simulink model "Control_v2"  (R2019b)
settings: Solver=FixedStepAuto  StartTime=0.0  StopTime=10  FixedStep=str2num(Step_size)  RelTol=1e-3
model workspace: external: MATLAB File H:\4-project\matlab\github\Sim-v2\bicopter_sim\Bicopter_DataFile14.m (data not in the file)
values from neighbouring files (symbols this model uses):
  b = [5,1,5,4]    [init_ADRC_val.m]    (also in init_Non_Linear_ADRC_val.m = 0.5*[1,    1, 6,  6]')
  b_sep = gains(5:8)    [get_ADRC_parameters.m]    (also in get_adrc_sep.m = [  2   7    6   7]; get_adrc_sep_kalman.m = [  2   2    6   7])
  C = [eye(4),zeros(4,8)]    [init_ADRC_val.m]
  C_air = 0.0025    [Sim_Script.m]
  d_f_phi = 100    [Sim_Script.m]
  d_f_psi = 25    [Sim_Script.m]
  d_f_theta = 10    [Sim_Script.m]
  d_f_z = 100    [Sim_Script.m]
  eps_sep = 0.7*[1 1 1 1]    [get_ADRC_parameters.m]    (also in get_adrc_sep.m = [0.7 0.3 0.3 0.35]; get_adrc_sep_kalman.m = [0.7 0.7 0.3 0.35])
  epsi = 1.5    [init_Non_Linear_ADRC_val.m]
  euler_source = 1    [Sim_Script.m]
  freq_cut_angvel_phi = 75    [Sim_Script.m]
  freq_cut_angvel_psi = 75    [Sim_Script.m]
  freq_cut_angvel_theta = 50    [Sim_Script.m]
  g = 9.81    [Sim_Script.m]
  K = place(A1,B1,w00(1:8))    [init_ADRC_val.m]
  L = place(A',C',8*w00)'    [init_ADRC_val.m]
  method = STSC_controller    (= 2)    [Sim_Script.m]
  method_angle_plane_sw = plane_sw    (= 2)    [Sim_Script.m]
  mult_obs = 10    [init_Non_Linear_ADRC_val.m]
  Noise_gain = 1    [Sim_Script.m]
  PID_VAL_SEP = init_pid_val_sep()    [Sim_Script.m]
  polarity = [-1;1;1;1]    [Sim_Script.m]
  r = [10,5,10,10]    [init_Non_Linear_ADRC_val.m]
  S_phi = 0.001    [Sim_Script.m]
  S_psi = S_phi    (= 0.001)    [Sim_Script.m]
  S_theta = S_phi    (= 0.001)    [Sim_Script.m]
  State_step = [Z_step;Phi_step;Theta_step;Psi_step]    [req_response.m]
  Step_size = step_size    [Sim_Script.m]
  STSC_VAL = init_STSC_val()    [Sim_Script.m]
  time_delay = 1e-6    (= 1e-06)    [Sim_Script.m]
  V_phi = 0.01    [Sim_Script.m]
  V_psi = 0.01    [Sim_Script.m]
  V_theta = 0.01    [Sim_Script.m]
  wc_sep = gains(1:4)    [get_ADRC_parameters.m]    (also in get_adrc_sep.m = [ 5.54   9   6    3]; get_adrc_sep_kalman.m = [ 5.54   9   6    3])
  wo_sep = ga*wc_sep    [get_ADRC_parameters.m]    (also in get_adrc_sep.m; get_adrc_sep_kalman.m)
undefined symbols (not defined in the file or in its folder): Continuous, magnitude, NLADRC_VAL, sigbuilder_block, smiData, Time, X, Y, Z
libraries: sm_lib x141, nesl_utility x20, simulink x19, fuzblock x3, sharedtransform x1, ctrlSharedLib x1
(part 5 of 7)

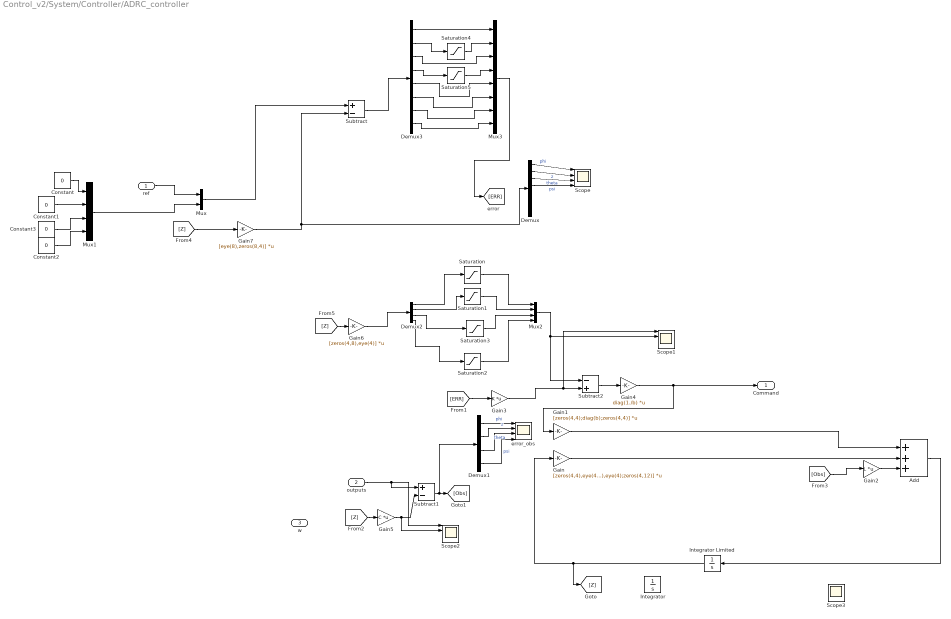
== system Control_v2/System/Controller/ADRC_controller ==
  ref : Inport
  outputs : Inport  Port=2
  w : Inport  Port=3
  Add : Sum  Inputs=+++
  Constant{,1..3} (4 alike) : Constant  Value=0
  Demux : Demux  Outputs=8
  Demux1 : Demux
  Demux2 : Demux
  Demux3 : Demux  Outputs=8
  Gain : Gain  Gain=[zeros(4,4),eye(4),zeros(4,4);zeros(4,4),zeros(4,4),eye(4);zeros(4,12)]  Multiplication=Matrix(K*u)
  Gain1 : Gain  Gain=[zeros(4,4);diag(b);zeros(4,4)]  Multiplication=Matrix(K*u)
  Gain2 : Gain  Gain=L  Multiplication=Matrix(K*u)
  Gain3 : Gain  Gain=K  Multiplication=Matrix(K*u)
  Gain4 : Gain  Gain=diag(1./b)  Multiplication=Matrix(K*u)
  Gain5 : Gain  Gain=C  Multiplication=Matrix(K*u)
  Gain6 : Gain  Gain=[zeros(4,8),eye(4)]  Multiplication=Matrix(K*u)
  Gain7 : Gain  Gain=[eye(8),zeros(8,4)]  Multiplication=Matrix(K*u)
  Integrator : Integrator  InitialCondition=zeros(12,1)
  Integrator Limited : Integrator  LimitOutput=on  UpperSaturationLimit=100  LowerSaturationLimit=-100
  Mux : Mux  Inputs=2
  Mux1 : Mux
  Mux2 : Mux
  Mux3 : Mux  Inputs=8
  Saturation : Saturate  UpperLimit=0.1  LowerLimit=-0.1
  Saturation1 : Saturate  UpperLimit=6  LowerLimit=-6
  Saturation2 : Saturate  UpperLimit=0.1  LowerLimit=-0.1
  Saturation3 : Saturate  UpperLimit=0.3  LowerLimit=-0.3
  Saturation4 : Saturate  UpperLimit=1  LowerLimit=-1
  Saturation5 : Saturate  UpperLimit=0.4  LowerLimit=-0.4
  Scope{,1..3} (4 alike) : Scope  NumInputPorts=4
  Subtract : Sum  Inputs=+-
  Subtract1 : Sum  Inputs=+-
  Subtract2 : Sum  Inputs=-+
  error_obs : Scope  NumInputPorts=4
  Command : Outport
  wires:
  Gain1/1 -> Add/1
  Gain3/1 -> Scope1/1, Subtract2/2
  Gain2/1 -> Add/3
  outputs/1 -> Scope2/1, Subtract1/1
  Gain5/1 -> Scope2/2, Subtract1/2
  Subtract1/1 -> Demux1/1, [Obs]
  Subtract2/1 -> Gain4/1
  Constant1/1 -> Mux1/2
  Constant/1 -> Mux1/1
  Constant3/1 -> Mux1/3
  Constant2/1 -> Mux1/4
  Mux1/1 -> Mux/2
  Mux/1 -> Subtract/1
  Gain4/1 -> Gain1/1, Command/1
  [Obs] -> Gain2/1
  [ERR] -> Gain3/1
  [Z] -> Gain5/1
  [Z] -> Gain7/1
  [Z] -> Gain6/1
  Demux/1 -> Scope/1  "phi"
  Demux/2 -> Scope/2  "z"
  Demux/3 -> Scope/3  "theta"
  Demux/4 -> Scope/4  "psi"
  Demux1/2 -> error_obs/2  "z"
  Demux1/1 -> error_obs/1  "phi"
  Demux1/4 -> error_obs/4  "psi"
  Demux1/3 -> error_obs/3  "theta"
  Add/1 -> Integrator Limited/1
  Integrator Limited/1 -> Gain/1, [Z]
  Gain/1 -> Add/2
  Saturation3/1 -> Mux2/3
  Saturation/1 -> Mux2/1
  Demux2/2 -> Saturation1/1
  Demux2/4 -> Saturation2/1
  Saturation1/1 -> Mux2/2
  Demux2/1 -> Saturation/1
  Demux2/3 -> Saturation3/1
  Saturation2/1 -> Mux2/4
  Gain6/1 -> Demux2/1
  Mux2/1 -> Subtract2/1, Scope1/2
  ref/1 -> Mux/1
  Gain7/1 -> Demux/1, Subtract/2
  Saturation5/1 -> Mux3/4
  Demux3/3 -> Mux3/3
  Demux3/4 -> Saturation5/1
  Saturation4/1 -> Mux3/2
  Demux3/1 -> Mux3/1
  Demux3/2 -> Saturation4/1
  Subtract/1 -> Demux3/1
  Demux3/5 -> Mux3/5
  Demux3/6 -> Mux3/6
  Demux3/7 -> Mux3/7
  Demux3/8 -> Mux3/8
  Mux3/1 -> [ERR]

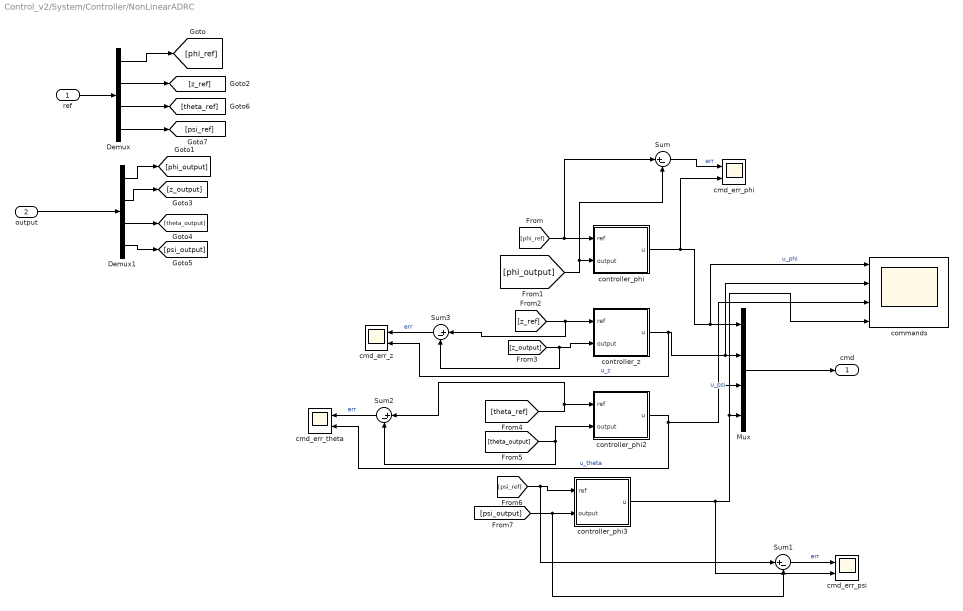
== system Control_v2/System/Controller/NonLinearADRC ==
  ref : Inport
  output : Inport  Port=2
  Demux : Demux
  Demux1 : Demux
  Mux : Mux
  Sum{,1..3} (4 alike) : Sum  Inputs=|+-
  cmd_err_phi : Scope  NumInputPorts=2
  cmd_err_psi : Scope  NumInputPorts=2
  cmd_err_theta : Scope  NumInputPorts=2
  cmd_err_z : Scope  NumInputPorts=2
  commands : Scope  NumInputPorts=4
  controller_phi : Subsystem  mask{ind=1}
      mask prompts: ind "index"
  controller_phi2 : Subsystem  mask{ind=3}
      mask prompts: ind "index"
  controller_phi3 : Subsystem  mask{ind=4}
      mask prompts: ind "index"
  controller_z : Subsystem  mask{ind=2}
      mask prompts: ind "index"
  cmd : Outport
  wires:
  ref/1 -> Demux/1
  output/1 -> Demux1/1
  Demux/1 -> [phi_ref]
  Demux1/1 -> [phi_output]
  Demux1/2 -> [z_output]
  Demux1/4 -> [psi_output]
  Demux1/3 -> [theta_output]
  Demux/2 -> [z_ref]
  Demux/3 -> [theta_ref]
  Demux/4 -> [psi_ref]
  [phi_ref] -> Sum/1, controller_phi/1(ref)
  [phi_output] -> Sum/2, controller_phi/2(output)
  [z_output] -> controller_z/2(output), Sum3/2
  [z_ref] -> controller_z/1(ref), Sum3/1
  [theta_output] -> controller_phi2/2(output), Sum2/2
  controller_phi/1(u) -> cmd_err_phi/2, commands/1, Mux/1  "u_phi"
  controller_z/1(u) -> cmd_err_z/2, commands/2, Mux/2  "u_z"
  controller_phi2/1(u) -> commands/3, Mux/3, cmd_err_theta/2  "u_theta"
  controller_phi3/1(u) -> cmd_err_psi/2, commands/4, Mux/4  "u_psi"
  Mux/1 -> cmd/1
  Sum/1 -> cmd_err_phi/1  "err"
  Sum1/1 -> cmd_err_psi/1  "err"
  [psi_ref] -> controller_phi3/1(ref), Sum1/1
  [psi_output] -> controller_phi3/2(output), Sum1/2
  Sum2/1 -> cmd_err_theta/1  "err"
  [theta_ref] -> controller_phi2/1(ref), Sum2/1
  Sum3/1 -> cmd_err_z/1  "err"

== system Control_v2/System/Controller/PID_Controller ==
  ref : Inport
  y : Inport  Port=2
  speed : Inport  Port=3
  Demux1 : Demux
  Demux2 : Demux
  Mux2 : Mux
  Saturation : Saturate  UpperLimit=2  LowerLimit=-2
  Saturation1 : Saturate  UpperLimit=0.6  LowerLimit=-0.6
  Sum : Sum  Inputs=|+-
  inner_loop1 : Subsystem  mask{parm_id=1, f=d_f_z}
  inner_loop2 : Subsystem  mask{parm_id=3, f=300}
  inner_loop4 : Subsystem  mask{parm_id=2, f=300}
  inner_loop7 : Subsystem  mask{parm_id=4, f=25}
  cmd : Outport
  wires:
  inner_loop1/1(cmd) -> Mux2/2
  inner_loop2/1(cmd) -> Mux2/3
  Demux1/1 -> inner_loop4/2(y_dot)
  Demux1/2 -> inner_loop1/2(y_dot)
  Demux2/2 -> Saturation/1
  Demux1/3 -> inner_loop2/2(y_dot)
  inner_loop4/1(cmd) -> Mux2/1
  inner_loop7/1(cmd) -> Mux2/4
  Mux2/1 -> cmd/1
  Sum/1 -> Demux2/1
  y/1 -> Sum/2
  speed/1 -> Demux1/1
  ref/1 -> Sum/1
  Demux1/4 -> inner_loop7/2(y_dot)
  Demux2/1 -> inner_loop4/1(err)
  Demux2/3 -> inner_loop2/1(err)
  Demux2/4 -> Saturation1/1
  Saturation/1 -> inner_loop1/1(err)
  Saturation1/1 -> inner_loop7/1(err)

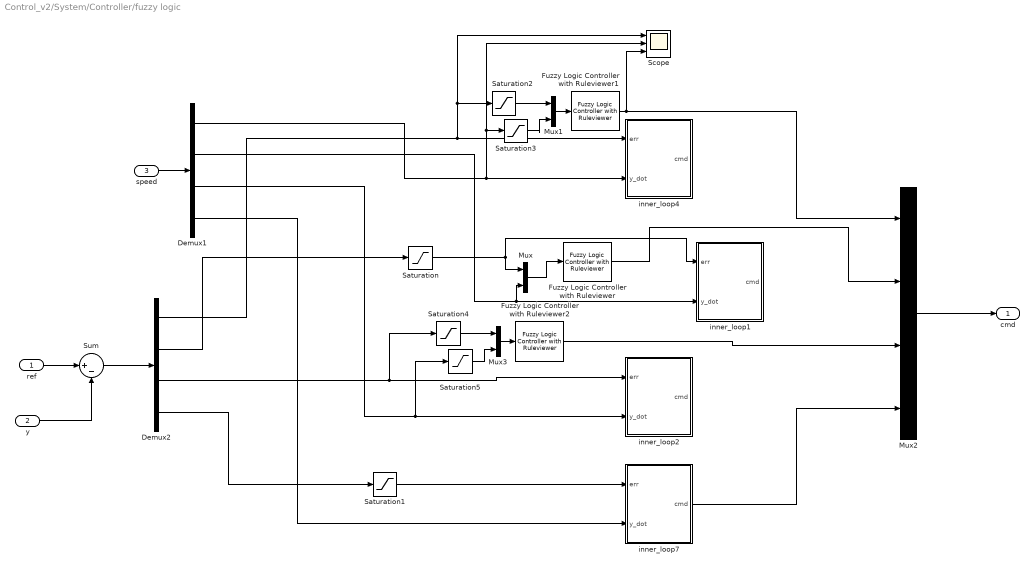
== system Control_v2/System/Controller/fuzzy logic ==
  ref : Inport
  y : Inport  Port=2
  speed : Inport  Port=3
  Demux1 : Demux
  Demux2 : Demux
  Fuzzy Logic Controller with Ruleviewer : fuzblock/Fuzzy Logic  Controller  with Ruleviewer  fismatrix=z_fuzzy  Ts=2
  Fuzzy Logic Controller with Ruleviewer1 : fuzblock/Fuzzy Logic  Controller  with Ruleviewer  fismatrix=phi_fuzzy  Ts=2
  Fuzzy Logic Controller with Ruleviewer2 : fuzblock/Fuzzy Logic  Controller  with Ruleviewer  fismatrix=theta_fuzzy  Ts=2
  Mux : Mux  Inputs=2
  Mux1 : Mux  Inputs=2
  Mux2 : Mux
  Mux3 : Mux  Inputs=2
  Saturation : Saturate  UpperLimit=1  LowerLimit=-1
  Saturation1 : Saturate  UpperLimit=0.4  LowerLimit=-0.4
  Saturation2 : Saturate
  Saturation3 : Saturate  UpperLimit=2  LowerLimit=-2
  Saturation4 : Saturate
  Saturation5 : Saturate  UpperLimit=2  LowerLimit=-2
  Scope : Scope  NumInputPorts=3
  Sum : Sum  Inputs=|+-
  inner_loop1 : Subsystem  mask{parm_id=1, f=d_f_z}
  inner_loop2 : Subsystem  mask{parm_id=3, f=d_f_theta}
  inner_loop4 : Subsystem  mask{parm_id=2, f=d_f_phi}
  inner_loop7 : Subsystem  mask{parm_id=4, f=d_f_psi}
  cmd : Outport
  wires:
  Demux1/1 -> Scope/2, Saturation3/1, inner_loop4/2(y_dot)
  Demux1/2 -> Mux/2, inner_loop1/2(y_dot)
  Demux2/2 -> Saturation/1
  Demux1/3 -> Saturation5/1, inner_loop2/2(y_dot)
  inner_loop7/1(cmd) -> Mux2/4
  Mux2/1 -> cmd/1
  Sum/1 -> Demux2/1
  y/1 -> Sum/2
  speed/1 -> Demux1/1
  ref/1 -> Sum/1
  Demux1/4 -> inner_loop7/2(y_dot)
  Demux2/1 -> Saturation2/1, Scope/1, inner_loop4/1(err)
  Demux2/3 -> Saturation4/1, inner_loop2/1(err)
  Demux2/4 -> Saturation1/1
  Saturation/1 -> Mux/1, inner_loop1/1(err)
  Saturation1/1 -> inner_loop7/1(err)
  Mux/1 -> Fuzzy Logic Controller with Ruleviewer/1
  Fuzzy Logic Controller with Ruleviewer/1 -> Mux2/2
  Mux1/1 -> Fuzzy Logic Controller with Ruleviewer1/1
  Fuzzy Logic Controller with Ruleviewer1/1 -> Scope/3, Mux2/1
  Saturation2/1 -> Mux1/1
  Saturation3/1 -> Mux1/2
  Saturation4/1 -> Mux3/1
  Saturation5/1 -> Mux3/2
  Mux3/1 -> Fuzzy Logic Controller with Ruleviewer2/1
  Fuzzy Logic Controller with Ruleviewer2/1 -> Mux2/3

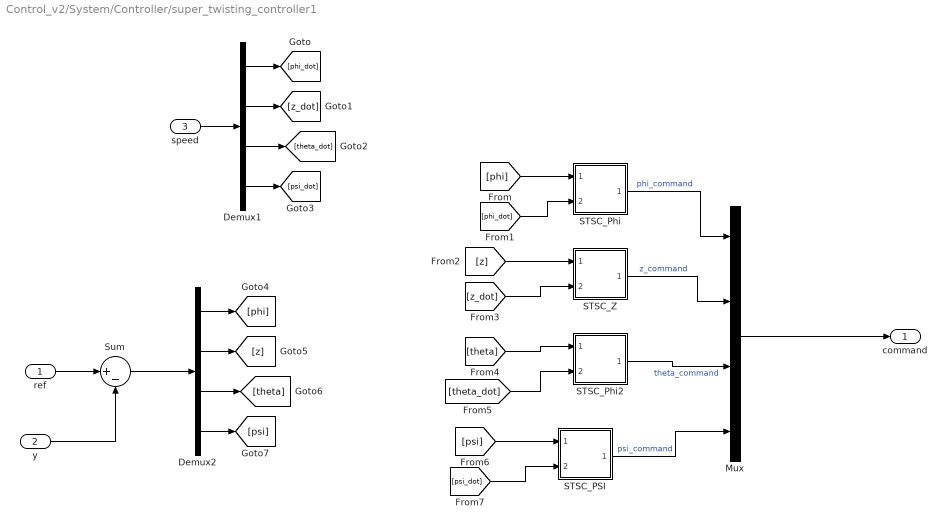
== system Control_v2/System/Controller/super_twisting_controller1 ==
  ref : Inport
  y : Inport  Port=2
  speed : Inport  Port=3
  Demux1 : Demux
  Demux2 : Demux
  Mux : Mux
  STSC_PSI : Subsystem  mask{parm_id=4, f=25}
  STSC_Phi : Subsystem  mask{parm_id=2, f=500}
  STSC_Phi2 : Subsystem  mask{parm_id=3, f=200}
  STSC_Z : Subsystem  mask{parm_id=1, f=500}
  Sum : Sum  Inputs=|+-
  command : Outport
  wires:
  STSC_Phi2/1(cmd) -> Mux/3  "theta_command"
  STSC_Phi/1(cmd) -> Mux/1  "phi_command"
  STSC_Z/1(cmd) -> Mux/2  "z_command"
  Mux/1 -> command/1
  STSC_PSI/1(cmd) -> Mux/4  "psi_command"
  speed/1 -> Demux1/1
  Demux1/4 -> [psi_dot]
  Demux1/3 -> [theta_dot]
  Demux1/2 -> [z_dot]
  Demux1/1 -> [phi_dot]
  Demux2/3 -> [theta]
  Demux2/4 -> [psi]
  Demux2/1 -> [phi]
  Demux2/2 -> [z]
  [psi_dot] -> STSC_PSI/2(error_dot)
  [phi] -> STSC_Phi/1(error)
  [phi_dot] -> STSC_Phi/2(error_dot)
  [z_dot] -> STSC_Z/2(error_dot)
  [z] -> STSC_Z/1(error)
  [theta] -> STSC_Phi2/1(error)
  [theta_dot] -> STSC_Phi2/2(error_dot)
  ref/1 -> Sum/1
  y/1 -> Sum/2
  Sum/1 -> Demux2/1
  [psi] -> STSC_PSI/1(error)

== system Control_v2/System/angvel_2_euler/Gyro low pass filter ==
  In1 : Inport
  Demux : Demux  Outputs=3
  Mux : Mux  Inputs=3
  Transfer Fcn : TransferFcn  Denominator=[1/(2*pi*freq_cut_angvel_phi) 1]
  Transfer Fcn1 : TransferFcn  Denominator=[1/(2*pi*freq_cut_angvel_theta) 1]
  Transfer Fcn2 : TransferFcn  Denominator=[1/(2*pi*freq_cut_angvel_psi) 1]
  Out1 : Outport
  wires:
  In1/1 -> Demux/1
  Mux/1 -> Out1/1
  Transfer Fcn2/1 -> Mux/3
  Transfer Fcn1/1 -> Mux/2
  Transfer Fcn/1 -> Mux/1
  Demux/1 -> Transfer Fcn/1
  Demux/2 -> Transfer Fcn1/1
  Demux/3 -> Transfer Fcn2/1

== system Control_v2/System/angvel_2_euler/noise ==
  Input : Inport
  Band-Limited White Noise : simulink/Sources/Band-Limited White Noise  Cov=[S_phi*V_phi]  Ts=S_phi  seed=[23341]
  Band-Limited White Noise1 : simulink/Sources/Band-Limited White Noise  Cov=[S_theta*V_theta]  Ts=S_theta  seed=[23341]
  Band-Limited White Noise2 : simulink/Sources/Band-Limited White Noise  Cov=[S_psi*V_psi]  Ts=S_psi  seed=[23341]
  Gain : Gain  Gain=Noise_gain
  Gain1 : Gain  Gain=0.1
  Mux : Mux  Inputs=3
  Mux1 : Mux  Inputs=2
  Scope : Scope
  Scope1 : Scope
  Out1 : Outport
  wires:
  Band-Limited White Noise/1 -> Mux/1
  Band-Limited White Noise1/1 -> Mux/2
  Mux/1 -> Gain/1
  Band-Limited White Noise2/1 -> Mux/3
  Gain/1 -> Scope1/1, Out1/1
  Input/1 -> Mux1/1, Gain1/1
  Gain1/1 -> Mux1/2
  Mux1/1 -> Scope/1

== system Control_v2/System/Bicopter/air_force/Subsystem ==
  fx : Inport
  fy : Inport  Port=2
  fz : Inport  Port=3
  External Force and Torque : sm_lib/Forces and Torques/External Force and Torque  ForceResolutionFrame=AttachedFrame  EnableForceX=on  EnableForceY=on  EnableForceZ=on  EnableForce=off  TorqueResolutionFrame=AttachedFrame  EnableTorqueX=off  EnableTorqueY=off  EnableTorqueZ=off  EnableTorque=off
  Gain : Gain
  Gain1 : Gain
  Gain2 : Gain
  Simulink-PS Converter : nesl_utility/Simulink-PS Converter  PhysicalDomain=network_engine_domain  SubClassName=ps_input  LeftPortType=input  RightPortType=output  PseudoPeriodic=off  Frequencies=[]  NoiseDistribution=none  NoiseParameters=[]  Unit=1  AffineConversion=off  FilteringAndDerivatives=provide  SimscapeFilterOrder=1  InputFilterTimeConstant=0.001  UdotUserProvided=0
  Simulink-PS Converter1 : nesl_utility/Simulink-PS Converter  PhysicalDomain=network_engine_domain  SubClassName=ps_input  LeftPortType=input  RightPortType=output  PseudoPeriodic=off  Frequencies=[]  NoiseDistribution=none  NoiseParameters=[]  Unit=1  AffineConversion=off  FilteringAndDerivatives=provide  SimscapeFilterOrder=1  InputFilterTimeConstant=0.001  UdotUserProvided=0
  Simulink-PS Converter2 : nesl_utility/Simulink-PS Converter  PhysicalDomain=network_engine_domain  SubClassName=ps_input  LeftPortType=input  RightPortType=output  PseudoPeriodic=off  Frequencies=[]  NoiseDistribution=none  NoiseParameters=[]  Unit=1  AffineConversion=off  FilteringAndDerivatives=provide  SimscapeFilterOrder=1  InputFilterTimeConstant=0.001  UdotUserProvided=0
  Conn1 : PMIOPort  Side=Right
  wires:
  fx/1 -> Gain/1
  Gain/1 -> Simulink-PS Converter/1
  Gain1/1 -> Simulink-PS Converter1/1
  fy/1 -> Gain1/1
  Gain2/1 -> Simulink-PS Converter2/1
  fz/1 -> Gain2/1
  connections:
  External Force and Torque/LConn1 -- Simulink-PS Converter/RConn1
  Conn1/RConn1 -- External Force and Torque/RConn1
  Simulink-PS Converter1/RConn1 -- External Force and Torque/LConn2
  Simulink-PS Converter2/RConn1 -- External Force and Torque/LConn3

== system Control_v2/System/Controller/ADRC_Kalman/Phi_loop ==
  ref : Inport
  y : Inport  Port=2
  Constant : Constant  Value=0
  Constant1 : Constant  Value=0
  Demux : Demux  Outputs=3
  Gain : Gain  Gain=wc_sep(ind)^2
  Gain1 : Gain  Gain=2*eps_sep(ind)*wc_sep(ind)
  Gain2 : Gain  Gain=1/b_sep(ind)
  Gain3 : Gain  Gain=0.1
  Kalman Filter : ctrlSharedLib/Kalman Filter  TimeDomain=Continuous-Time  UseCurrentEstimator=on  ModelSource=Individual A, B, C, D matrices  ModelSourceVariable=ss(0.95,1,1,0,1)  A=[0 1 0; 0 0 1; 0 0 0]  B=[0;b_sep(ind);0]  C=[1 0 0]  D=0  NumberOfStates=1  NumberOfInputs=1  NumberOfOutputs=1  InitialEstimateSource=Dialog  X0=[0 0 0]  P0=10  UseK=off  UseGH=on  NumberOfProcessNoiseInputs=1  G=[1;1;10]  TimeInvariantG=on  H=0  TimeInvariantH=on  Q=0.0001  TimeInvariantQ=on  R=0.0001  TimeInvariantR=on  N=0  TimeInvariantN=on  AddInputPort=on  AddEnablePort=off  OutputEstimatedY=off  OutputP=off  Ts=-1
      settings: SourceProductBaseCode=CT
  LESO : Subsystem
  MATLAB Function : MATLAB Function  TreatAsAtomicUnit=on
  Mux : Mux  Inputs=3
  Saturation : Saturate  UpperLimit=0.3  LowerLimit=-0.3
  Scope : Scope  NumInputPorts=2
  Scope1 : Scope  NumInputPorts=6
  Sum : Sum  Inputs=|+-
  Sum1 : Sum  Inputs=|+-
  Sum2 : Sum  Inputs=|+-
  Output : Outport
  wires:
  ref/1 -> Sum/1  "err"
  Gain/1 -> Scope1/2, Sum1/1
  Gain1/1 -> Sum1/2, Scope1/3
  Sum1/1 -> Scope1/4, Sum2/1
  Sum2/1 -> Scope1/5, Gain2/1
  Gain2/1 -> Kalman Filter/1, Scope1/6, Output/1
  y/1 -> Kalman Filter/2, Scope/2, LESO/1(y)  "err"
  LESO/3(Z3) -> Gain3/1
  Kalman Filter/1 -> Demux/1
  Demux/3 -> Sum2/2
  Demux/2 -> Gain1/1
  Sum/1 -> Scope1/1, Gain/1
  Constant/1 -> Mux/1
  Constant1/1 -> Mux/3
  Demux/1 -> Sum/2, Scope/1

== system Control_v2/System/Controller/ADRC_Kalman/Z_loop ==
  ref : Inport
  y : Inport  Port=2
  Gain : Gain  Gain=wc_sep(ind)^2
  Gain1 : Gain  Gain=2*eps_sep(ind)*wc_sep(ind)
  Gain2 : Gain  Gain=1/b_sep(ind)
  LESO : Subsystem
  Saturation : Saturate  UpperLimit=0.6  LowerLimit=-0.6
  Sum : Sum  Inputs=|+-
  Sum1 : Sum  Inputs=|+-
  Sum2 : Sum  Inputs=|+-
  Output : Outport
  wires:
  y/1 -> LESO/1(y)  "err"
  Gain2/1 -> Output/1
  Sum2/1 -> Gain2/1, LESO/2(u)
  LESO/3(Z3) -> Sum2/2
  Sum1/1 -> Sum2/1
  Gain1/1 -> Sum1/2
  Gain/1 -> Sum1/1
  Sum/1 -> Saturation/1
  ref/1 -> Sum/1  "err"
  LESO/1(Z1) -> Sum/2
  LESO/2(Z2) -> Gain1/1
  Saturation/1 -> Gain/1

== system Control_v2/System/Controller/ADRC_Kalman/psi_loop ==
  ref : Inport
  y : Inport  Port=2
  Gain : Gain  Gain=wc_sep(ind)^2
  Gain1 : Gain  Gain=2*eps_sep(ind)*wc_sep(ind)
  Gain2 : Gain  Gain=1/b_sep(ind)
  Gain3 : Gain  Gain=0.4
  LESO : Subsystem
  Saturation : Saturate  UpperLimit=0.3  LowerLimit=-0.3
  Sum : Sum  Inputs=|+-
  Sum1 : Sum  Inputs=|+-
  Sum2 : Sum  Inputs=|+-
  Output : Outport
  wires:
  y/1 -> LESO/1(y)  "err"
  Gain2/1 -> Output/1
  Sum2/1 -> Gain2/1, LESO/2(u)
  Sum1/1 -> Sum2/1
  Gain1/1 -> Sum1/2
  Gain/1 -> Sum1/1
  Sum/1 -> Saturation/1
  ref/1 -> Sum/1  "err"
  LESO/1(Z1) -> Sum/2
  LESO/2(Z2) -> Gain1/1
  Gain3/1 -> Sum2/2
  Saturation/1 -> Gain/1
  LESO/3(Z3) -> Gain3/1

== system Control_v2/System/Controller/ADRC_Kalman/theta_loop ==
  ref : Inport
  y : Inport  Port=2
  Gain : Gain  Gain=wc_sep(ind)^2
  Gain1 : Gain  Gain=2*eps_sep(ind)*wc_sep(ind)
  Gain2 : Gain  Gain=1/b_sep(ind)
  Gain3 : Gain  Gain=0.02
  LESO : Subsystem
  Sum : Sum  Inputs=|+-
  Sum1 : Sum  Inputs=|+-
  Sum2 : Sum  Inputs=|+-
  Output : Outport
  wires:
  LESO/2(Z2) -> Gain1/1
  LESO/1(Z1) -> Sum/2
  ref/1 -> Sum/1  "err"
  Sum/1 -> Gain/1
  Gain/1 -> Sum1/1
  Gain1/1 -> Sum1/2
  Sum1/1 -> Sum2/1
  Sum2/1 -> LESO/2(u), Gain2/1
  Gain2/1 -> Output/1
  y/1 -> LESO/1(y)  "err"
  Gain3/1 -> Sum2/2
  LESO/3(Z3) -> Gain3/1

== system Control_v2/System/Controller/ADRC_SEP/Phi_loop ==
  ref : Inport
  y : Inport  Port=2
  Gain : Gain  Gain=wc_sep(ind)^2
  Gain1 : Gain  Gain=2*eps_sep(ind)*wc_sep(ind)
  Gain2 : Gain  Gain=1/b_sep(ind)
  Gain3 : Gain  Gain=0.1
  LESO : Subsystem
  Saturation : Saturate  UpperLimit=0.3  LowerLimit=-0.3
  Scope : Scope  NumInputPorts=2
  Scope1 : Scope  NumInputPorts=5
  Sum : Sum  Inputs=|+-
  Sum1 : Sum  Inputs=|+-
  Sum2 : Sum  Inputs=|+-
  Output : Outport
  wires:
  LESO/2(Z2) -> Gain1/1
  LESO/1(Z1) -> Scope/1, Sum/2
  ref/1 -> Sum/1  "err"
  Gain/1 -> Scope1/2, Sum1/1
  Gain1/1 -> Sum1/2, Scope1/3
  Sum1/1 -> Scope1/4, Sum2/1
  Sum2/1 -> Scope1/5, LESO/2(u), Gain2/1
  Gain2/1 -> Output/1
  y/1 -> Scope/2, LESO/1(y)  "err"
  LESO/3(Z3) -> Gain3/1
  Sum/1 -> Saturation/1
  Gain3/1 -> Sum2/2
  Saturation/1 -> Scope1/1, Gain/1

== system Control_v2/System/Controller/ADRC_SEP/Z_loop ==
  ref : Inport
  y : Inport  Port=2
  Gain : Gain  Gain=wc_sep(ind)^2
  Gain1 : Gain  Gain=2*eps_sep(ind)*wc_sep(ind)
  Gain2 : Gain  Gain=1/b_sep(ind)
  LESO : Subsystem
  Saturation : Saturate  UpperLimit=0.6  LowerLimit=-0.6
  Sum : Sum  Inputs=|+-
  Sum1 : Sum  Inputs=|+-
  Sum2 : Sum  Inputs=|+-
  Output : Outport
  wires:
  y/1 -> LESO/1(y)  "err"
  Gain2/1 -> Output/1
  Sum2/1 -> Gain2/1, LESO/2(u)
  LESO/3(Z3) -> Sum2/2
  Sum1/1 -> Sum2/1
  Gain1/1 -> Sum1/2
  Gain/1 -> Sum1/1
  Sum/1 -> Saturation/1
  ref/1 -> Sum/1  "err"
  LESO/1(Z1) -> Sum/2
  LESO/2(Z2) -> Gain1/1
  Saturation/1 -> Gain/1

== system Control_v2/System/Controller/ADRC_SEP/psi_loop ==
  ref : Inport
  y : Inport  Port=2
  Gain : Gain  Gain=wc_sep(ind)^2
  Gain1 : Gain  Gain=2*eps_sep(ind)*wc_sep(ind)
  Gain2 : Gain  Gain=1/b_sep(ind)
  Gain3 : Gain  Gain=0.4
  LESO : Subsystem
  Saturation : Saturate  UpperLimit=0.3  LowerLimit=-0.3
  Sum : Sum  Inputs=|+-
  Sum1 : Sum  Inputs=|+-
  Sum2 : Sum  Inputs=|+-
  Output : Outport
  wires:
  y/1 -> LESO/1(y)  "err"
  Gain2/1 -> Output/1
  Sum2/1 -> Gain2/1, LESO/2(u)
  Sum1/1 -> Sum2/1
  Gain1/1 -> Sum1/2
  Gain/1 -> Sum1/1
  Sum/1 -> Saturation/1
  ref/1 -> Sum/1  "err"
  LESO/1(Z1) -> Sum/2
  LESO/2(Z2) -> Gain1/1
  Gain3/1 -> Sum2/2
  Saturation/1 -> Gain/1
  LESO/3(Z3) -> Gain3/1

== system Control_v2/System/Controller/ADRC_SEP/theta_loop ==
  ref : Inport
  y : Inport  Port=2
  Gain : Gain  Gain=wc_sep(ind)^2
  Gain1 : Gain  Gain=2*eps_sep(ind)*wc_sep(ind)
  Gain2 : Gain  Gain=1/b_sep(ind)
  Gain3 : Gain  Gain=0.02
  LESO : Subsystem
  Sum : Sum  Inputs=|+-
  Sum1 : Sum  Inputs=|+-
  Sum2 : Sum  Inputs=|+-
  Output : Outport
  wires:
  LESO/2(Z2) -> Gain1/1
  LESO/1(Z1) -> Sum/2
  ref/1 -> Sum/1  "err"
  Sum/1 -> Gain/1
  Gain/1 -> Sum1/1
  Gain1/1 -> Sum1/2
  Sum1/1 -> Sum2/1
  Sum2/1 -> LESO/2(u), Gain2/1
  Gain2/1 -> Output/1
  y/1 -> LESO/1(y)  "err"
  Gain3/1 -> Sum2/2
  LESO/3(Z3) -> Gain3/1

== system Control_v2/System/Controller/NonLinearADRC/controller_phi ==
  ref : Inport
  output : Inport  Port=2
  1/b : Gain  Gain=1/NLADRC_VAL(ind,4)
  Derivative : Derivative
  ESO : Subsystem
  NLSEF : Subsystem
  Scope : Scope  NumInputPorts=2
  Scope{1..4} (4 alike) : Scope
  Scope6 : Scope  NumInputPorts=2
  Sum : Sum  Inputs=|+-
  Sum1 : Sum  Inputs=|+-
  Sum2 : Sum  Inputs=|+-
  TD : Subsystem
  b : Gain  Gain=NLADRC_VAL(ind,4)
  phi : Scope  NumInputPorts=2
  u : Outport
  wires:
  Sum1/1 -> NLSEF/2(e2)
  Sum/1 -> Scope2/1, NLSEF/1(e1)
  b/1 -> ESO/2(b*u)
  ESO/3(Z1) -> Sum/2, Scope/1  "Z1"
  ESO/2(Z2) -> Sum1/2
  TD/2(Z2) -> Scope6/1, Sum1/1  "Z2"
  output/1 -> Scope/2, ESO/1(y)  "output"
  NLSEF/1(u) -> Scope3/1, Sum2/1
  Sum2/1 -> 1/b/1
  ref/1 -> phi/1, Derivative/1, TD/1(v0)  "ref"
  TD/1(Z1) -> phi/2, Sum/1  "Z1"
  ESO/1(Z3) -> Sum2/2, Scope1/1
  Derivative/1 -> Scope6/2  "der"
  1/b/1 -> b/1, u/1

== system Control_v2/System/Controller/NonLinearADRC/controller_phi2 ==
  ref : Inport
  output : Inport  Port=2
  1/b : Gain  Gain=1/NLADRC_VAL(ind,4)
  Derivative : Derivative
  ESO : Subsystem
  NLSEF : Subsystem
  Scope : Scope  NumInputPorts=2
  Scope{1..4} (4 alike) : Scope
  Scope6 : Scope  NumInputPorts=2
  Sum : Sum  Inputs=|+-
  Sum1 : Sum  Inputs=|+-
  Sum2 : Sum  Inputs=|+-
  TD : Subsystem
  b : Gain  Gain=NLADRC_VAL(ind,4)
  phi : Scope  NumInputPorts=2
  u : Outport
  wires:
  Sum1/1 -> NLSEF/2(e2)
  Sum/1 -> Scope2/1, NLSEF/1(e1)
  b/1 -> ESO/2(b*u)
  ESO/3(Z1) -> Sum/2, Scope/1  "Z1"
  ESO/2(Z2) -> Sum1/2
  TD/2(Z2) -> Scope6/1, Sum1/1  "Z2"
  output/1 -> Scope/2, ESO/1(y)  "output"
  NLSEF/1(u) -> Scope3/1, Sum2/1
  Sum2/1 -> 1/b/1
  ref/1 -> phi/1, Derivative/1, TD/1(v0)  "ref"
  TD/1(Z1) -> phi/2, Sum/1  "Z1"
  ESO/1(Z3) -> Sum2/2, Scope1/1
  Derivative/1 -> Scope6/2  "der"
  1/b/1 -> b/1, u/1

== system Control_v2/System/Controller/NonLinearADRC/controller_phi3 ==
  ref : Inport
  output : Inport  Port=2
  1/b : Gain  Gain=1/NLADRC_VAL(ind,4)
  Derivative : Derivative
  ESO : Subsystem
  NLSEF : Subsystem
  Scope : Scope  NumInputPorts=2
  Scope{1..4} (4 alike) : Scope
  Scope6 : Scope  NumInputPorts=2
  Sum : Sum  Inputs=|+-
  Sum1 : Sum  Inputs=|+-
  Sum2 : Sum  Inputs=|+-
  TD : Subsystem
  b : Gain  Gain=NLADRC_VAL(ind,4)
  phi : Scope  NumInputPorts=2
  u : Outport
  wires:
  1/b/1 -> u/1, b/1
  Derivative/1 -> Scope6/2  "der"
  ESO/1(Z3) -> Sum2/2, Scope1/1
  TD/1(Z1) -> Sum/1, phi/2  "Z1"
  ref/1 -> TD/1(v0), Derivative/1, phi/1  "ref"
  Sum2/1 -> 1/b/1
  NLSEF/1(u) -> Sum2/1, Scope3/1
  output/1 -> ESO/1(y), Scope/2  "output"
  TD/2(Z2) -> Sum1/1, Scope6/1  "Z2"
  ESO/2(Z2) -> Sum1/2
  ESO/3(Z1) -> Sum/2, Scope/1  "Z1"
  b/1 -> ESO/2(b*u)
  Sum/1 -> NLSEF/1(e1), Scope2/1
  Sum1/1 -> NLSEF/2(e2)

== system Control_v2/System/Controller/NonLinearADRC/controller_z ==
  ref : Inport
  output : Inport  Port=2
  1/b : Gain  Gain=1/NLADRC_VAL(ind,4)
  Derivative : Derivative
  ESO : Subsystem
  NLSEF : Subsystem
  Scope : Scope  NumInputPorts=2
  Scope{1..4} (4 alike) : Scope
  Scope6 : Scope  NumInputPorts=2
  Sum : Sum  Inputs=|+-
  Sum1 : Sum  Inputs=|+-
  Sum2 : Sum  Inputs=|+-
  TD : Subsystem
  b : Gain  Gain=NLADRC_VAL(ind,4)
  phi : Scope  NumInputPorts=2
  u : Outport
  wires:
  1/b/1 -> u/1, b/1
  Derivative/1 -> Scope6/2  "der"
  ESO/1(Z3) -> Sum2/2, Scope1/1
  TD/1(Z1) -> Sum/1, phi/2  "Z1"
  ref/1 -> TD/1(v0), Derivative/1, phi/1  "ref"
  Sum2/1 -> 1/b/1
  NLSEF/1(u) -> Sum2/1, Scope3/1
  output/1 -> ESO/1(y), Scope/2  "output"
  TD/2(Z2) -> Sum1/1, Scope6/1  "Z2"
  ESO/2(Z2) -> Sum1/2
  ESO/3(Z1) -> Sum/2, Scope/1  "Z1"
  b/1 -> ESO/2(b*u)
  Sum/1 -> NLSEF/1(e1), Scope2/1
  Sum1/1 -> Scope4/1, NLSEF/2(e2)

== system Control_v2/System/Controller/PID_Controller/inner_loop1 ==
  note: Scope_P
  err : Inport
  y_dot : Inport  Port=2
  Derivative : Derivative
  Gain : Gain  Gain=PID_VAL_SEP(parm_id,3)
  Gain1 : Gain  Gain=PID_VAL_SEP(parm_id,3)
  Gain2 : Gain  Gain=PID_VAL_SEP(parm_id,2)
  I : simulink/Continuous/PID Controller  Controller=PID  Form=Parallel  TimeDomain=Continuous-time  SampleTime=-1  IntegratorMethod=Forward Euler  FilterMethod=Forward Euler  ControllerParametersSource=internal  P=0  I=PID_VAL_SEP(parm_id,2)  D=0  UseFilter=on  N=0  TunerSelectOption=Transfer Function Based (PID Tuner App)  InitialConditionSource=internal  InitialConditionForIntegrator=0  InitialConditionForFilter=0  DifferentiatorICPrevScaledInput=0  ExternalReset=none  TrackingMode=off  Kt=1  LimitOutput=off  UpperSaturationLimit=inf  LowerSaturationLimit=-inf  LinearizeAsGain=on  AntiWindupMode=none  Kb=1  POutMin=[]  POutMax=[]  IOutMin=[]  IOutMax=[]  DOutMin=[]  DOutMax=[]  NOutMin=[]  NOutMax=[]  SumOutMin=[]  SumOutMax=[]  SaturationOutMin=[]  SaturationOutMax=[]  PParamMin=[]  PParamMax=[]  IParamMin=[]  IParamMax=[]  DParamMin=[]  DParamMax=[]  NParamMin=[]  NParamMax=[]  KbParamMin=[]  KbParamMax=[]  KtParamMin=[]  KtParamMax=[]  KbOutMin=[]  KbOutMax=[]  KtOutMin=[]  KtOutMax=[]  IntegratorOutMin=[]  IntegratorOutMax=[]  FilterOutMin=[]  FilterOutMax=[]  SumI1OutMin=[]  SumI1OutMax=[]  SumI2OutMin=[]  SumI2OutMax=[]  SumI3OutMin=[]  SumI3OutMax=[]  SumI4OutMin=[]  SumI4OutMax=[]  SumDOutMin=[]  SumDOutMax=[]  DifferentiatorOutMin=[]  DifferentiatorOutMax=[]  FilterDiffOutCoefMin=[]  FilterDiffOutCoefMax=[]  ReciprocalOutMin=[]  ReciprocalOutMax=[]  SumDenOutMin=[]  SumDenOutMax=[]  SumNumOutMin=[]  SumNumOutMax=[]  DivideOutMin=[]  DivideOutMax=[]  IntegratorContinuousStateAttributes=''  IntegratorStateMustResolveToSignalObject=off  IntegratorRTWStateStorageClass=Auto  FilterContinuousStateAttributes=''  FilterStateMustResolveToSignalObject=off  FilterRTWStateStorageClass=Auto  ParallelPVariant=InternalParameters  IdealPVariant=Disabled  IVariant=InternalParameters  DVariant=InternalParameters  IntegratorVariant=Continuous  SatVariant=Disabled  AWVariant=Passthrough  PCopyVariant=Disabled  TRVariant=Disabled  FdbkBlocksVariant=Forward  IdealPFdbkVariant=Disabled  SatFdbkVariant=Disabled  DerivativeFilterVariant=ContFilter  NVariant=InternalParameters  NCopyVariant=Disabled  FilterICVariant=InternalICsFilter  IntegratorICVariant=InternalICs  ExternalResetVariant=Disabled  TRSumVariant=Passthrough  SumFdbkVariant=Disabled  SumVariant=Sum_PID
  Integrator Limited : Integrator  LimitOutput=on  UpperSaturationLimit=5  LowerSaturationLimit=-5
  P : simulink/Continuous/PID Controller  Controller=PID  Form=Parallel  TimeDomain=Continuous-time  SampleTime=-1  IntegratorMethod=Forward Euler  FilterMethod=Forward Euler  ControllerParametersSource=internal  P=PID_VAL_SEP(parm_id,1)  I=0  D=0  UseFilter=on  N=0  TunerSelectOption=Transfer Function Based (PID Tuner App)  InitialConditionSource=internal  InitialConditionForIntegrator=0  InitialConditionForFilter=0  DifferentiatorICPrevScaledInput=0  ExternalReset=none  TrackingMode=off  Kt=1  LimitOutput=off  UpperSaturationLimit=inf  LowerSaturationLimit=-inf  LinearizeAsGain=on  AntiWindupMode=none  Kb=1  POutMin=[]  POutMax=[]  IOutMin=[]  IOutMax=[]  DOutMin=[]  DOutMax=[]  NOutMin=[]  NOutMax=[]  SumOutMin=[]  SumOutMax=[]  SaturationOutMin=[]  SaturationOutMax=[]  PParamMin=[]  PParamMax=[]  IParamMin=[]  IParamMax=[]  DParamMin=[]  DParamMax=[]  NParamMin=[]  NParamMax=[]  KbParamMin=[]  KbParamMax=[]  KtParamMin=[]  KtParamMax=[]  KbOutMin=[]  KbOutMax=[]  KtOutMin=[]  KtOutMax=[]  IntegratorOutMin=[]  IntegratorOutMax=[]  FilterOutMin=[]  FilterOutMax=[]  SumI1OutMin=[]  SumI1OutMax=[]  SumI2OutMin=[]  SumI2OutMax=[]  SumI3OutMin=[]  SumI3OutMax=[]  SumI4OutMin=[]  SumI4OutMax=[]  SumDOutMin=[]  SumDOutMax=[]  DifferentiatorOutMin=[]  DifferentiatorOutMax=[]  FilterDiffOutCoefMin=[]  FilterDiffOutCoefMax=[]  ReciprocalOutMin=[]  ReciprocalOutMax=[]  SumDenOutMin=[]  SumDenOutMax=[]  SumNumOutMin=[]  SumNumOutMax=[]  DivideOutMin=[]  DivideOutMax=[]  IntegratorContinuousStateAttributes=''  IntegratorStateMustResolveToSignalObject=off  IntegratorRTWStateStorageClass=Auto  FilterContinuousStateAttributes=''  FilterStateMustResolveToSignalObject=off  FilterRTWStateStorageClass=Auto  ParallelPVariant=InternalParameters  IdealPVariant=Disabled  IVariant=InternalParameters  DVariant=InternalParameters  IntegratorVariant=Continuous  SatVariant=Disabled  AWVariant=Passthrough  PCopyVariant=Disabled  TRVariant=Disabled  FdbkBlocksVariant=Forward  IdealPFdbkVariant=Disabled  SatFdbkVariant=Disabled  DerivativeFilterVariant=ContFilter  NVariant=InternalParameters  NCopyVariant=Disabled  FilterICVariant=InternalICsFilter  IntegratorICVariant=InternalICs  ExternalResetVariant=Disabled  TRSumVariant=Passthrough  SumFdbkVariant=Disabled  SumVariant=Sum_PID
  Scope : Scope  NumInputPorts=2
  Scope1 : Scope  NumInputPorts=2
  Scope_D : Scope  NumInputPorts=2
  Scope_D1 : Scope  NumInputPorts=2
  Scope_I : Scope  NumInputPorts=2
  Sum : Sum  Inputs=|+++-
  Transfer Fcn : TransferFcn  Numerator=[2*pi*f]  Denominator=[1 2*pi*f]
  Transfer Fcn1 : TransferFcn  Numerator=[2*pi*f]  Denominator=[1 2*pi*f]
  phiCmd : Scope  NumInputPorts=2
  cmd : Outport
  wires:
  Sum/1 -> phiCmd/2, cmd/1  "after"
  y_dot/1 -> Transfer Fcn1/1, Scope_D/1
  err/1 -> Gain2/1, Gain1/1, I/1, Scope_I/2, P/1, Scope/1, phiCmd/1  "err"
  P/1 -> Sum/1, Scope/2
  I/1 -> Scope1/2, Scope_I/1
  Gain1/1 -> Derivative/1  "before"
  Derivative/1 -> Transfer Fcn/1
  Gain/1 -> Sum/4  "before"
  Gain2/1 -> Integrator Limited/1
  Integrator Limited/1 -> Scope1/1, Sum/3
  Transfer Fcn1/1 -> Gain/1  "after"

== system Control_v2/System/Controller/PID_Controller/inner_loop2 ==
  note: Scope_P
  err : Inport
  y_dot : Inport  Port=2
  Derivative : Derivative
  Gain : Gain  Gain=PID_VAL_SEP(parm_id,3)
  Gain1 : Gain  Gain=PID_VAL_SEP(parm_id,3)
  I : simulink/Continuous/PID Controller  Controller=PID  Form=Parallel  TimeDomain=Continuous-time  SampleTime=-1  IntegratorMethod=Forward Euler  FilterMethod=Forward Euler  ControllerParametersSource=internal  P=0  I=PID_VAL_SEP(parm_id,2)  D=0  UseFilter=on  N=0  TunerSelectOption=Transfer Function Based (PID Tuner App)  InitialConditionSource=internal  InitialConditionForIntegrator=0  InitialConditionForFilter=0  DifferentiatorICPrevScaledInput=0  ExternalReset=none  TrackingMode=off  Kt=1  LimitOutput=off  UpperSaturationLimit=inf  LowerSaturationLimit=-inf  LinearizeAsGain=on  AntiWindupMode=none  Kb=1  POutMin=[]  POutMax=[]  IOutMin=[]  IOutMax=[]  DOutMin=[]  DOutMax=[]  NOutMin=[]  NOutMax=[]  SumOutMin=[]  SumOutMax=[]  SaturationOutMin=[]  SaturationOutMax=[]  PParamMin=[]  PParamMax=[]  IParamMin=[]  IParamMax=[]  DParamMin=[]  DParamMax=[]  NParamMin=[]  NParamMax=[]  KbParamMin=[]  KbParamMax=[]  KtParamMin=[]  KtParamMax=[]  KbOutMin=[]  KbOutMax=[]  KtOutMin=[]  KtOutMax=[]  IntegratorOutMin=[]  IntegratorOutMax=[]  FilterOutMin=[]  FilterOutMax=[]  SumI1OutMin=[]  SumI1OutMax=[]  SumI2OutMin=[]  SumI2OutMax=[]  SumI3OutMin=[]  SumI3OutMax=[]  SumI4OutMin=[]  SumI4OutMax=[]  SumDOutMin=[]  SumDOutMax=[]  DifferentiatorOutMin=[]  DifferentiatorOutMax=[]  FilterDiffOutCoefMin=[]  FilterDiffOutCoefMax=[]  ReciprocalOutMin=[]  ReciprocalOutMax=[]  SumDenOutMin=[]  SumDenOutMax=[]  SumNumOutMin=[]  SumNumOutMax=[]  DivideOutMin=[]  DivideOutMax=[]  IntegratorContinuousStateAttributes=''  IntegratorStateMustResolveToSignalObject=off  IntegratorRTWStateStorageClass=Auto  FilterContinuousStateAttributes=''  FilterStateMustResolveToSignalObject=off  FilterRTWStateStorageClass=Auto  ParallelPVariant=InternalParameters  IdealPVariant=Disabled  IVariant=InternalParameters  DVariant=InternalParameters  IntegratorVariant=Continuous  SatVariant=Disabled  AWVariant=Passthrough  PCopyVariant=Disabled  TRVariant=Disabled  FdbkBlocksVariant=Forward  IdealPFdbkVariant=Disabled  SatFdbkVariant=Disabled  DerivativeFilterVariant=ContFilter  NVariant=InternalParameters  NCopyVariant=Disabled  FilterICVariant=InternalICsFilter  IntegratorICVariant=InternalICs  ExternalResetVariant=Disabled  TRSumVariant=Passthrough  SumFdbkVariant=Disabled  SumVariant=Sum_PID
  P : simulink/Continuous/PID Controller  Controller=PID  Form=Parallel  TimeDomain=Continuous-time  SampleTime=-1  IntegratorMethod=Forward Euler  FilterMethod=Forward Euler  ControllerParametersSource=internal  P=PID_VAL_SEP(parm_id,1)  I=0  D=0  UseFilter=on  N=0  TunerSelectOption=Transfer Function Based (PID Tuner App)  InitialConditionSource=internal  InitialConditionForIntegrator=0  InitialConditionForFilter=0  DifferentiatorICPrevScaledInput=0  ExternalReset=none  TrackingMode=off  Kt=1  LimitOutput=off  UpperSaturationLimit=inf  LowerSaturationLimit=-inf  LinearizeAsGain=on  AntiWindupMode=none  Kb=1  POutMin=[]  POutMax=[]  IOutMin=[]  IOutMax=[]  DOutMin=[]  DOutMax=[]  NOutMin=[]  NOutMax=[]  SumOutMin=[]  SumOutMax=[]  SaturationOutMin=[]  SaturationOutMax=[]  PParamMin=[]  PParamMax=[]  IParamMin=[]  IParamMax=[]  DParamMin=[]  DParamMax=[]  NParamMin=[]  NParamMax=[]  KbParamMin=[]  KbParamMax=[]  KtParamMin=[]  KtParamMax=[]  KbOutMin=[]  KbOutMax=[]  KtOutMin=[]  KtOutMax=[]  IntegratorOutMin=[]  IntegratorOutMax=[]  FilterOutMin=[]  FilterOutMax=[]  SumI1OutMin=[]  SumI1OutMax=[]  SumI2OutMin=[]  SumI2OutMax=[]  SumI3OutMin=[]  SumI3OutMax=[]  SumI4OutMin=[]  SumI4OutMax=[]  SumDOutMin=[]  SumDOutMax=[]  DifferentiatorOutMin=[]  DifferentiatorOutMax=[]  FilterDiffOutCoefMin=[]  FilterDiffOutCoefMax=[]  ReciprocalOutMin=[]  ReciprocalOutMax=[]  SumDenOutMin=[]  SumDenOutMax=[]  SumNumOutMin=[]  SumNumOutMax=[]  DivideOutMin=[]  DivideOutMax=[]  IntegratorContinuousStateAttributes=''  IntegratorStateMustResolveToSignalObject=off  IntegratorRTWStateStorageClass=Auto  FilterContinuousStateAttributes=''  FilterStateMustResolveToSignalObject=off  FilterRTWStateStorageClass=Auto  ParallelPVariant=InternalParameters  IdealPVariant=Disabled  IVariant=InternalParameters  DVariant=InternalParameters  IntegratorVariant=Continuous  SatVariant=Disabled  AWVariant=Passthrough  PCopyVariant=Disabled  TRVariant=Disabled  FdbkBlocksVariant=Forward  IdealPFdbkVariant=Disabled  SatFdbkVariant=Disabled  DerivativeFilterVariant=ContFilter  NVariant=InternalParameters  NCopyVariant=Disabled  FilterICVariant=InternalICsFilter  IntegratorICVariant=InternalICs  ExternalResetVariant=Disabled  TRSumVariant=Passthrough  SumFdbkVariant=Disabled  SumVariant=Sum_PID
  Scope : Scope  NumInputPorts=2
  Scope_D : Scope  NumInputPorts=2
  Scope_D1 : Scope  NumInputPorts=2
  Scope_I : Scope  NumInputPorts=2
  Sum : Sum  Inputs=|+++-
  Transfer Fcn : TransferFcn  Numerator=[2*pi*f]  Denominator=[1 2*pi*f]
  Transfer Fcn1 : TransferFcn  Numerator=[2*pi*f]  Denominator=[1 2*pi*f]
  phiCmd : Scope  NumInputPorts=2
  cmd : Outport
  wires:
  Gain/1 -> Scope_D1/2, Sum/4  "before"
  I/1 -> Scope_I/1, Sum/2
  P/1 -> Scope/2, Sum/1
  err/1 -> phiCmd/1, Gain1/1, Scope/1, P/1, Scope_I/2, I/1  "err"
  Sum/1 -> cmd/1, phiCmd/2  "after"
  Gain1/1 -> Derivative/1  "before"
  Transfer Fcn/1 -> Scope_D/1  "after"
  y_dot/1 -> Transfer Fcn1/1  "after"
  Transfer Fcn1/1 -> Gain/1  "after"

== system Control_v2/System/Controller/PID_Controller/inner_loop4 ==
  note: Scope_P
  err : Inport
  y_dot : Inport  Port=2
  Derivative : Derivative
  Gain : Gain  Gain=PID_VAL_SEP(parm_id,3)
  Gain1 : Gain  Gain=PID_VAL_SEP(parm_id,3)
  I : simulink/Continuous/PID Controller  Controller=PID  Form=Parallel  TimeDomain=Continuous-time  SampleTime=-1  IntegratorMethod=Forward Euler  FilterMethod=Forward Euler  ControllerParametersSource=internal  P=0  I=PID_VAL_SEP(parm_id,2)  D=0  UseFilter=on  N=0  TunerSelectOption=Transfer Function Based (PID Tuner App)  InitialConditionSource=internal  InitialConditionForIntegrator=0  InitialConditionForFilter=0  DifferentiatorICPrevScaledInput=0  ExternalReset=none  TrackingMode=off  Kt=1  LimitOutput=off  UpperSaturationLimit=inf  LowerSaturationLimit=-inf  LinearizeAsGain=on  AntiWindupMode=none  Kb=1  POutMin=[]  POutMax=[]  IOutMin=[]  IOutMax=[]  DOutMin=[]  DOutMax=[]  NOutMin=[]  NOutMax=[]  SumOutMin=[]  SumOutMax=[]  SaturationOutMin=[]  SaturationOutMax=[]  PParamMin=[]  PParamMax=[]  IParamMin=[]  IParamMax=[]  DParamMin=[]  DParamMax=[]  NParamMin=[]  NParamMax=[]  KbParamMin=[]  KbParamMax=[]  KtParamMin=[]  KtParamMax=[]  KbOutMin=[]  KbOutMax=[]  KtOutMin=[]  KtOutMax=[]  IntegratorOutMin=[]  IntegratorOutMax=[]  FilterOutMin=[]  FilterOutMax=[]  SumI1OutMin=[]  SumI1OutMax=[]  SumI2OutMin=[]  SumI2OutMax=[]  SumI3OutMin=[]  SumI3OutMax=[]  SumI4OutMin=[]  SumI4OutMax=[]  SumDOutMin=[]  SumDOutMax=[]  DifferentiatorOutMin=[]  DifferentiatorOutMax=[]  FilterDiffOutCoefMin=[]  FilterDiffOutCoefMax=[]  ReciprocalOutMin=[]  ReciprocalOutMax=[]  SumDenOutMin=[]  SumDenOutMax=[]  SumNumOutMin=[]  SumNumOutMax=[]  DivideOutMin=[]  DivideOutMax=[]  IntegratorContinuousStateAttributes=''  IntegratorStateMustResolveToSignalObject=off  IntegratorRTWStateStorageClass=Auto  FilterContinuousStateAttributes=''  FilterStateMustResolveToSignalObject=off  FilterRTWStateStorageClass=Auto  ParallelPVariant=InternalParameters  IdealPVariant=Disabled  IVariant=InternalParameters  DVariant=InternalParameters  IntegratorVariant=Continuous  SatVariant=Disabled  AWVariant=Passthrough  PCopyVariant=Disabled  TRVariant=Disabled  FdbkBlocksVariant=Forward  IdealPFdbkVariant=Disabled  SatFdbkVariant=Disabled  DerivativeFilterVariant=ContFilter  NVariant=InternalParameters  NCopyVariant=Disabled  FilterICVariant=InternalICsFilter  IntegratorICVariant=InternalICs  ExternalResetVariant=Disabled  TRSumVariant=Passthrough  SumFdbkVariant=Disabled  SumVariant=Sum_PID
  P : simulink/Continuous/PID Controller  Controller=PID  Form=Parallel  TimeDomain=Continuous-time  SampleTime=-1  IntegratorMethod=Forward Euler  FilterMethod=Forward Euler  ControllerParametersSource=internal  P=PID_VAL_SEP(parm_id,1)  I=0  D=0  UseFilter=on  N=0  TunerSelectOption=Transfer Function Based (PID Tuner App)  InitialConditionSource=internal  InitialConditionForIntegrator=0  InitialConditionForFilter=0  DifferentiatorICPrevScaledInput=0  ExternalReset=none  TrackingMode=off  Kt=1  LimitOutput=off  UpperSaturationLimit=inf  LowerSaturationLimit=-inf  LinearizeAsGain=on  AntiWindupMode=none  Kb=1  POutMin=[]  POutMax=[]  IOutMin=[]  IOutMax=[]  DOutMin=[]  DOutMax=[]  NOutMin=[]  NOutMax=[]  SumOutMin=[]  SumOutMax=[]  SaturationOutMin=[]  SaturationOutMax=[]  PParamMin=[]  PParamMax=[]  IParamMin=[]  IParamMax=[]  DParamMin=[]  DParamMax=[]  NParamMin=[]  NParamMax=[]  KbParamMin=[]  KbParamMax=[]  KtParamMin=[]  KtParamMax=[]  KbOutMin=[]  KbOutMax=[]  KtOutMin=[]  KtOutMax=[]  IntegratorOutMin=[]  IntegratorOutMax=[]  FilterOutMin=[]  FilterOutMax=[]  SumI1OutMin=[]  SumI1OutMax=[]  SumI2OutMin=[]  SumI2OutMax=[]  SumI3OutMin=[]  SumI3OutMax=[]  SumI4OutMin=[]  SumI4OutMax=[]  SumDOutMin=[]  SumDOutMax=[]  DifferentiatorOutMin=[]  DifferentiatorOutMax=[]  FilterDiffOutCoefMin=[]  FilterDiffOutCoefMax=[]  ReciprocalOutMin=[]  ReciprocalOutMax=[]  SumDenOutMin=[]  SumDenOutMax=[]  SumNumOutMin=[]  SumNumOutMax=[]  DivideOutMin=[]  DivideOutMax=[]  IntegratorContinuousStateAttributes=''  IntegratorStateMustResolveToSignalObject=off  IntegratorRTWStateStorageClass=Auto  FilterContinuousStateAttributes=''  FilterStateMustResolveToSignalObject=off  FilterRTWStateStorageClass=Auto  ParallelPVariant=InternalParameters  IdealPVariant=Disabled  IVariant=InternalParameters  DVariant=InternalParameters  IntegratorVariant=Continuous  SatVariant=Disabled  AWVariant=Passthrough  PCopyVariant=Disabled  TRVariant=Disabled  FdbkBlocksVariant=Forward  IdealPFdbkVariant=Disabled  SatFdbkVariant=Disabled  DerivativeFilterVariant=ContFilter  NVariant=InternalParameters  NCopyVariant=Disabled  FilterICVariant=InternalICsFilter  IntegratorICVariant=InternalICs  ExternalResetVariant=Disabled  TRSumVariant=Passthrough  SumFdbkVariant=Disabled  SumVariant=Sum_PID
  Scope : Scope  NumInputPorts=2
  Scope_D : Scope  NumInputPorts=2
  Scope_D1 : Scope  NumInputPorts=2
  Scope_I : Scope  NumInputPorts=2
  Sum : Sum  Inputs=|+++-
  Transfer Fcn : TransferFcn  Numerator=[2*pi*f]  Denominator=[1 2*pi*f]
  Transfer Fcn1 : TransferFcn  Numerator=[2*pi*f]  Denominator=[1 2*pi*f]
  phiCmd : Scope  NumInputPorts=2
  cmd : Outport
  wires:
  Gain/1 -> Sum/4, Scope_D1/2  "before"
  I/1 -> Scope_I/1, Sum/2
  P/1 -> Scope/2, Sum/1
  err/1 -> Gain1/1, Scope/1, P/1, Scope_I/2, I/1, phiCmd/1  "err"
  Sum/1 -> cmd/1, phiCmd/2  "after"
  Derivative/1 -> Scope_D/2, Transfer Fcn/1
  Gain1/1 -> Derivative/1  "before"
  Transfer Fcn/1 -> Scope_D/1  "after"
  y_dot/1 -> Transfer Fcn1/1  "after"
  Transfer Fcn1/1 -> Gain/1  "after"

== system Control_v2/System/Controller/PID_Controller/inner_loop7 ==
  note: Scope_P
  err : Inport
  y_dot : Inport  Port=2
  Derivative : Derivative
  Gain : Gain  Gain=PID_VAL_SEP(parm_id,3)
  Gain1 : Gain  Gain=PID_VAL_SEP(parm_id,3)
  Gain2 : Gain  Gain=PID_VAL_SEP(parm_id,2)
  I : simulink/Continuous/PID Controller  Controller=PID  Form=Parallel  TimeDomain=Continuous-time  SampleTime=-1  IntegratorMethod=Forward Euler  FilterMethod=Forward Euler  ControllerParametersSource=internal  P=0  I=PID_VAL_SEP(parm_id,2)  D=0  UseFilter=on  N=100  TunerSelectOption=Transfer Function Based (PID Tuner App)  InitialConditionSource=internal  InitialConditionForIntegrator=0  InitialConditionForFilter=0  DifferentiatorICPrevScaledInput=0  ExternalReset=none  TrackingMode=off  Kt=1  LimitOutput=off  UpperSaturationLimit=inf  LowerSaturationLimit=-inf  LinearizeAsGain=on  AntiWindupMode=none  Kb=1  POutMin=[]  POutMax=[]  IOutMin=[]  IOutMax=[]  DOutMin=[]  DOutMax=[]  NOutMin=[]  NOutMax=[]  SumOutMin=[]  SumOutMax=[]  SaturationOutMin=[]  SaturationOutMax=[]  PParamMin=[]  PParamMax=[]  IParamMin=[]  IParamMax=[]  DParamMin=[]  DParamMax=[]  NParamMin=[]  NParamMax=[]  KbParamMin=[]  KbParamMax=[]  KtParamMin=[]  KtParamMax=[]  KbOutMin=[]  KbOutMax=[]  KtOutMin=[]  KtOutMax=[]  IntegratorOutMin=[]  IntegratorOutMax=[]  FilterOutMin=[]  FilterOutMax=[]  SumI1OutMin=[]  SumI1OutMax=[]  SumI2OutMin=[]  SumI2OutMax=[]  SumI3OutMin=[]  SumI3OutMax=[]  SumI4OutMin=[]  SumI4OutMax=[]  SumDOutMin=[]  SumDOutMax=[]  DifferentiatorOutMin=[]  DifferentiatorOutMax=[]  FilterDiffOutCoefMin=[]  FilterDiffOutCoefMax=[]  ReciprocalOutMin=[]  ReciprocalOutMax=[]  SumDenOutMin=[]  SumDenOutMax=[]  SumNumOutMin=[]  SumNumOutMax=[]  DivideOutMin=[]  DivideOutMax=[]  IntegratorContinuousStateAttributes=''  IntegratorStateMustResolveToSignalObject=off  IntegratorRTWStateStorageClass=Auto  FilterContinuousStateAttributes=''  FilterStateMustResolveToSignalObject=off  FilterRTWStateStorageClass=Auto  ParallelPVariant=InternalParameters  IdealPVariant=Disabled  IVariant=InternalParameters  DVariant=InternalParameters  IntegratorVariant=Continuous  SatVariant=Disabled  AWVariant=Passthrough  PCopyVariant=Disabled  TRVariant=Disabled  FdbkBlocksVariant=Forward  IdealPFdbkVariant=Disabled  SatFdbkVariant=Disabled  DerivativeFilterVariant=ContFilter  NVariant=InternalParameters  NCopyVariant=Disabled  FilterICVariant=InternalICsFilter  IntegratorICVariant=InternalICs  ExternalResetVariant=Disabled  TRSumVariant=Passthrough  SumFdbkVariant=Disabled  SumVariant=Sum_PID
  Integrator Limited : Integrator  LimitOutput=on  UpperSaturationLimit=0.5  LowerSaturationLimit=-0.5
  P : simulink/Continuous/PID Controller  Controller=PID  Form=Parallel  TimeDomain=Continuous-time  SampleTime=-1  IntegratorMethod=Forward Euler  FilterMethod=Forward Euler  ControllerParametersSource=internal  P=PID_VAL_SEP(parm_id,1)  I=0  D=0  UseFilter=on  N=100  TunerSelectOption=Transfer Function Based (PID Tuner App)  InitialConditionSource=internal  InitialConditionForIntegrator=0  InitialConditionForFilter=0  DifferentiatorICPrevScaledInput=0  ExternalReset=none  TrackingMode=off  Kt=1  LimitOutput=off  UpperSaturationLimit=inf  LowerSaturationLimit=-inf  LinearizeAsGain=on  AntiWindupMode=none  Kb=1  POutMin=[]  POutMax=[]  IOutMin=[]  IOutMax=[]  DOutMin=[]  DOutMax=[]  NOutMin=[]  NOutMax=[]  SumOutMin=[]  SumOutMax=[]  SaturationOutMin=[]  SaturationOutMax=[]  PParamMin=[]  PParamMax=[]  IParamMin=[]  IParamMax=[]  DParamMin=[]  DParamMax=[]  NParamMin=[]  NParamMax=[]  KbParamMin=[]  KbParamMax=[]  KtParamMin=[]  KtParamMax=[]  KbOutMin=[]  KbOutMax=[]  KtOutMin=[]  KtOutMax=[]  IntegratorOutMin=[]  IntegratorOutMax=[]  FilterOutMin=[]  FilterOutMax=[]  SumI1OutMin=[]  SumI1OutMax=[]  SumI2OutMin=[]  SumI2OutMax=[]  SumI3OutMin=[]  SumI3OutMax=[]  SumI4OutMin=[]  SumI4OutMax=[]  SumDOutMin=[]  SumDOutMax=[]  DifferentiatorOutMin=[]  DifferentiatorOutMax=[]  FilterDiffOutCoefMin=[]  FilterDiffOutCoefMax=[]  ReciprocalOutMin=[]  ReciprocalOutMax=[]  SumDenOutMin=[]  SumDenOutMax=[]  SumNumOutMin=[]  SumNumOutMax=[]  DivideOutMin=[]  DivideOutMax=[]  IntegratorContinuousStateAttributes=''  IntegratorStateMustResolveToSignalObject=off  IntegratorRTWStateStorageClass=Auto  FilterContinuousStateAttributes=''  FilterStateMustResolveToSignalObject=off  FilterRTWStateStorageClass=Auto  ParallelPVariant=InternalParameters  IdealPVariant=Disabled  IVariant=InternalParameters  DVariant=InternalParameters  IntegratorVariant=Continuous  SatVariant=Disabled  AWVariant=Passthrough  PCopyVariant=Disabled  TRVariant=Disabled  FdbkBlocksVariant=Forward  IdealPFdbkVariant=Disabled  SatFdbkVariant=Disabled  DerivativeFilterVariant=ContFilter  NVariant=InternalParameters  NCopyVariant=Disabled  FilterICVariant=InternalICsFilter  IntegratorICVariant=InternalICs  ExternalResetVariant=Disabled  TRSumVariant=Passthrough  SumFdbkVariant=Disabled  SumVariant=Sum_PID
  Scope : Scope  NumInputPorts=2
  Scope1 : Scope  NumInputPorts=2
  Scope2 : Scope  NumInputPorts=4
  Scope_D : Scope  NumInputPorts=2
  Scope_D1 : Scope  NumInputPorts=2
  Scope_I : Scope  NumInputPorts=2
  Sum : Sum  Inputs=|+++-
  Sum1 : Sum  Inputs=|+-
  Transfer Fcn : TransferFcn  Numerator=[2*pi*f]  Denominator=[1 2*pi*f]
  Transfer Fcn1 : TransferFcn  Numerator=[2*pi*f]  Denominator=[1 2*pi*f]
  cmd : Outport
  wires:
  I/1 -> Scope_I/1
  P/1 -> Scope/2, Scope2/1, Sum/1
  err/1 -> Gain2/1, Gain1/1, Sum1/1
  Sum1/1 -> Scope1/1, Scope/1, P/1, Scope_I/2, I/1
  Gain/1 -> Sum/4, Scope_D1/2  "before"
  Sum/1 -> Scope2/4, Scope1/2, cmd/1  "after"
  y_dot/1 -> Transfer Fcn1/1, Scope_D/1  "after"
  Gain1/1 -> Derivative/1  "before"
  Derivative/1 -> Transfer Fcn/1
  Gain2/1 -> Integrator Limited/1
  Integrator Limited/1 -> Scope2/2, Sum/3
  Transfer Fcn1/1 -> Gain/1  "after"
